simulink model "abs_pid"  (R2020b)
settings: Solver=VariableStepAuto  StartTime=0.0  StopTime=50  RelTol=1e-3
undefined symbols (not defined in the file): A, c1, c2, c3, c4, Cd, d, F, H, J, kd, ki, kp, m, r, Tb, Vx, W, w
libraries: pid_lib x1
settings Model: Creator=K E S SRINIVAS  LastModifiedBy=K E S SRINIVAS

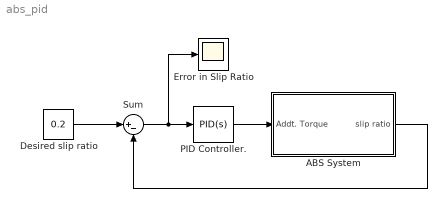
== system abs_pid ==
  ABS System : Subsystem
  Desired slip ratio : Constant  Value=0.2
  Error in Slip Ratio : Scope
  PID Controller. : pid_lib/PID Controller  Controller=PID  Form=Parallel  TimeDomain=Continuous-time  UseExternalTs=off  SampleTime=-1  IntegratorMethod=Forward Euler  FilterMethod=Forward Euler  ControllerParametersSource=internal  P=kp  I=ki  D=kd  UseFilter=on  N=100  TunerSelectOption=Transfer Function Based (PID Tuner App)  InitialConditionSource=internal  InitialConditionForIntegrator=0  InitialConditionForFilter=0  DifferentiatorICPrevScaledInput=0  ExternalReset=none  TrackingMode=off  Kt=1  LimitOutput=off  SatLimitsSource=internal  UpperSaturationLimit=inf  LowerSaturationLimit=-inf  LinearizeAsGain=on  AntiWindupMode=none  Kb=1  POutMin=[]  POutMax=[]  IOutMin=[]  IOutMax=[]  DOutMin=[]  DOutMax=[]  NOutMin=[]  NOutMax=[]  SumOutMin=[]  SumOutMax=[]  SaturationOutMin=[]  SaturationOutMax=[]  PParamMin=[]  PParamMax=[]  IParamMin=[]  IParamMax=[]  DParamMin=[]  DParamMax=[]  NParamMin=[]  NParamMax=[]  KbParamMin=[]  KbParamMax=[]  KtParamMin=[]  KtParamMax=[]  KbOutMin=[]  KbOutMax=[]  KtOutMin=[]  KtOutMax=[]  IntegratorOutMin=[]  IntegratorOutMax=[]  FilterOutMin=[]  FilterOutMax=[]  SumI1OutMin=[]  SumI1OutMax=[]  SumI2OutMin=[]  SumI2OutMax=[]  SumI3OutMin=[]  SumI3OutMax=[]  SumI4OutMin=[]  SumI4OutMax=[]  SumDOutMin=[]  SumDOutMax=[]  DifferentiatorOutMin=[]  DifferentiatorOutMax=[]  FilterDiffOutCoefMin=[]  FilterDiffOutCoefMax=[]  ReciprocalOutMin=[]  ReciprocalOutMax=[]  SumDenOutMin=[]  SumDenOutMax=[]  SumNumOutMin=[]  SumNumOutMax=[]  DivideOutMin=[]  DivideOutMax=[]  UdiffTsProdOutMin=[]  UdiffTsProdOutMax=[]  NTsProdOutMin=[]  NTsProdOutMax=[]  UintegralTsProdOutMin=[]  UintegralTsProdOutMax=[]  UngainTsProdOutMin=[]  UngainTsProdOutMax=[]  IntegratorContinuousStateAttributes=''  IntegratorStateMustResolveToSignalObject=off  IntegratorRTWStateStorageClass=Auto  FilterContinuousStateAttributes=''  FilterStateMustResolveToSignalObject=off  FilterRTWStateStorageClass=Auto  ParallelPVariant=InternalParameters  IdealPVariant=Disabled  IVariant=InternalParameters  DVariant=InternalParameters  IntegratorVariant=Continuous  SatVariant=Disabled  AWVariant=Passthrough  PCopyVariant=Disabled  TRVariant=Disabled  FdbkBlocksVariant=Forward  IdealPFdbkVariant=Disabled  SatFdbkVariant=Disabled  DerivativeFilterVariant=ContFilter  NVariant=InternalParameters  NCopyVariant=Disabled  FilterICVariant=InternalICsFilter  IntegratorICVariant=InternalICs  ExternalResetVariant=Disabled  TRSumVariant=Passthrough  SumFdbkVariant=Disabled  SumVariant=Sum_PID  TsampFilterVariant=InternalTs  TsampNgainVariant=Passthrough  TsampIntegralVariant=Passthrough  ExternalSaturationOutDataTypeStr=Inherit: Same as second input
  Sum : Sum  Inputs=|+-
  wires:
  ABS System/1(slip ratio) -> Sum/2
  Desired slip ratio/1 -> Sum/1
  PID Controller./1 -> ABS System/1(Addt. Torque)
  Sum/1 -> Error in Slip Ratio/1, PID Controller./1

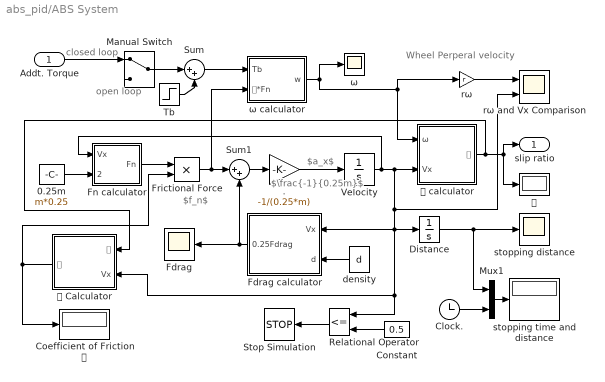
== system abs_pid/ABS System ==
  note: $a_x$
  note: $\frac{-1}{0.25m}$
  note: $f_n$
  note: Wheel Perperal velocity
  note: closed loop
  note: open loop
  Addt. Torque : Inport
  . : Gain  Gain=-1/(0.25*m)
  0.25m : Constant  Value=m*0.25
  Clock. : Clock
  Coefficient of Friction 𝜇 : Display
  Constant : Constant  Value=0.5
  Distance : Integrator
  Fdrag : Scope
  Fdrag calculator : Subsystem
  Fn calculator : Subsystem
  Frictional Force : Product
  Manual Switch : ManualSwitch
  Mux1 : Mux  Inputs=2
  Relational Operator : RelationalOperator  Operator=<=  OutDataTypeStr=boolean  RndMeth=Simplest
  Stop Simulation : Stop
  Sum : Sum  Inputs=|++
  Sum1 : Sum  Inputs=|++
  Tb : Step  Time=0  After=Tb  SampleTime=0
  Velocity : Integrator  InitialCondition=Vx  LimitOutput=on  LowerSaturationLimit=0
  density : Constant  Value=d
  rω : Gain  Gain=r
  "rω and Vx Comparison " : Scope  NumInputPorts=2
  stopping distance : Scope
  stopping time and distance : Display
  ω : Scope
  ω calculator : Subsystem
  𝜆 : Display
  𝜆 calculator : Subsystem
  𝜇 Calculator : Subsystem
  slip ratio : Outport
  wires:
  𝜇 Calculator/1(𝜇) -> Coefficient of Friction 𝜇/1, Frictional Force/2
  Velocity/1 -> 𝜆 calculator/2(Vx), Fdrag calculator/1(Vx), 𝜇 Calculator/2(Vx), Relational Operator/1, Distance/1, "rω and Vx Comparison "/2, Fn calculator/1(Vx)
  ./1 -> Velocity/1
  Relational Operator/1 -> Stop Simulation/1
  Constant/1 -> Relational Operator/2
  Sum/1 -> ω calculator/1(Tb)
  Addt. Torque/1 -> Manual Switch/1
  Tb/1 -> Sum/2
  ω calculator/1(w) -> rω/1, 𝜆 calculator/1(ω), ω/1
  𝜆 calculator/1(𝜆) -> slip ratio/1, 𝜆/1, 𝜇 Calculator/1(𝜆)
  Distance/1 -> stopping distance/1, Mux1/1
  rω/1 -> "rω and Vx Comparison "/1
  Mux1/1 -> stopping time and distance/1
  Manual Switch/1 -> Sum/1
  Sum1/1 -> ./1
  Fdrag calculator/1(0.25Fdrag) -> Sum1/2, Fdrag/1
  Frictional Force/1 -> Sum1/1, ω calculator/2(𝜇*Fn)
  Fn calculator/1(Fn) -> Frictional Force/1
  density/1 -> Fdrag calculator/2(d)
  0.25m/1 -> Fn calculator/2(0.25m)
  Clock./1 -> Mux1/2

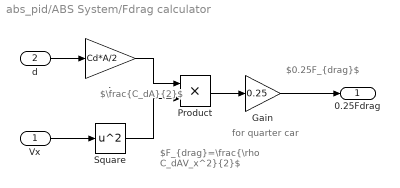
== system abs_pid/ABS System/Fdrag calculator ==
  note: $0.25F_{drag}$
  note: for quarter car
  note: $F_{drag}=\frac{\rho C_dAV_x^2}{2}$
  note: $\frac{C_dA}{2}$
  Vx : Inport
  d : Inport  Port=2
  . : Gain  Gain=Cd*A/2
  Gain : Gain  Gain=0.25
  Product : Product
  Square : Math  Operator=square  SaturateOnIntegerOverflow=on
  0.25Fdrag : Outport
  wires:
  Square/1 -> Product/2
  d/1 -> ./1
  ./1 -> Product/1
  Product/1 -> Gain/1
  Vx/1 -> Square/1
  Gain/1 -> 0.25Fdrag/1

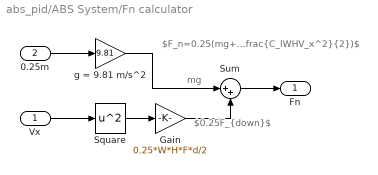
== system abs_pid/ABS System/Fn calculator ==
  note: mg
  note: $0.25F_{down}$
  note: $F_n=0.25(mg+\frac{C_lWHV_x^2}{2})$
  Vx : Inport
  0.25m : Inport  Port=2
  Gain : Gain  Gain=0.25*W*H*F*d/2
  Square : Math  Operator=square  SaturateOnIntegerOverflow=on
  Sum : Sum  Inputs=|++
  g = 9.81 m/s^2 : Gain  Gain=9.81
  Fn : Outport
  wires:
  Vx/1 -> Square/1
  Square/1 -> Gain/1
  Sum/1 -> Fn/1
  Gain/1 -> Sum/2
  0.25m/1 -> g = 9.81 m/s^2/1
  g = 9.81 m/s^2/1 -> Sum/1

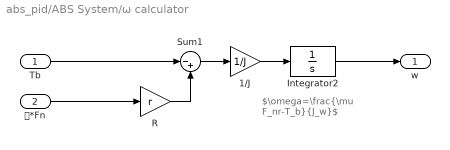
== system abs_pid/ABS System/ω calculator ==
  note: $\omega=\frac{\mu F_nr-T_b}{J_w}$
  Tb : Inport
  𝜇*Fn : Inport  Port=2
  1/J : Gain  Gain=1/J
  Integrator2 : Integrator  InitialCondition=w  LimitOutput=on  LowerSaturationLimit=0
  R : Gain  Gain=r
  Sum1 : Sum  Inputs=|-+
  w : Outport
  wires:
  Sum1/1 -> 1/J/1
  Tb/1 -> Sum1/1
  Integrator2/1 -> w/1
  𝜇*Fn/1 -> R/1
  1/J/1 -> Integrator2/1
  R/1 -> Sum1/2

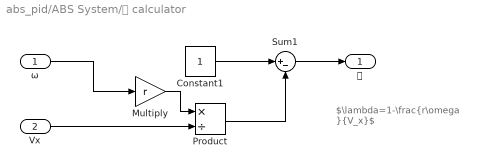
== system abs_pid/ABS System/𝜆 calculator ==
  note: $\lambda=1-\frac{r\omega }{V_x}$
  ω : Inport
  Vx : Inport  Port=2
  Constant1 : Constant
  Multiply : Gain  Gain=r
  Product : Product  Inputs=*/
  Sum1 : Sum  Inputs=|+-
  𝜆 : Outport
  wires:
  ω/1 -> Multiply/1
  Constant1/1 -> Sum1/1
  Vx/1 -> Product/2
  Multiply/1 -> Product/1
  Product/1 -> Sum1/2
  Sum1/1 -> 𝜆/1

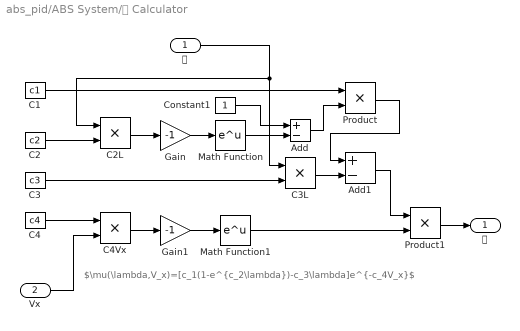
== system abs_pid/ABS System/𝜇 Calculator ==
  note: $\mu(\lambda,V_x)=[c_1(1-e^{c_2\lambda})-c_3\lambda]e^{-c_4V_x}$
  𝜆 : Inport
  Vx : Inport  Port=2
  Add : Sum  Inputs=+-
  Add1 : Sum  Inputs=+-
  C1 : Constant  Value=c1
  C2 : Constant  Value=c2
  C2L : Product
  C3 : Constant  Value=c3
  C3L : Product
  C4 : Constant  Value=c4
  C4Vx : Product
  Constant1 : Constant
  Gain : Gain  Gain=-1
  Gain1 : Gain  Gain=-1
  Math Function : Math  SaturateOnIntegerOverflow=on
  Math Function1 : Math  SaturateOnIntegerOverflow=on
  Product : Product
  Product1 : Product
  𝜇 : Outport
  wires:
  C2/1 -> C2L/2
  Gain/1 -> Math Function/1
  C1/1 -> Product/1
  C2L/1 -> Gain/1
  Constant1/1 -> Add/1
  Vx/1 -> C4Vx/2
  C4/1 -> C4Vx/1
  Add/1 -> Product/2
  Math Function/1 -> Add/2
  Gain1/1 -> Math Function1/1
  Math Function1/1 -> Product1/2
  C3L/1 -> Add1/2
  𝜆/1 -> C3L/1, C2L/1
  C4Vx/1 -> Gain1/1
  C3/1 -> C3L/2
  Product/1 -> Add1/1
  Add1/1 -> Product1/1
  Product1/1 -> 𝜇/1
